simulink model "pendule"  (R2023a)
settings: Solver=VariableStepAuto  StartTime=0.0  StopTime=10.0  RelTol=1e-3
settings Model: Creator=gwr2526  LastModifiedBy=gwr2526

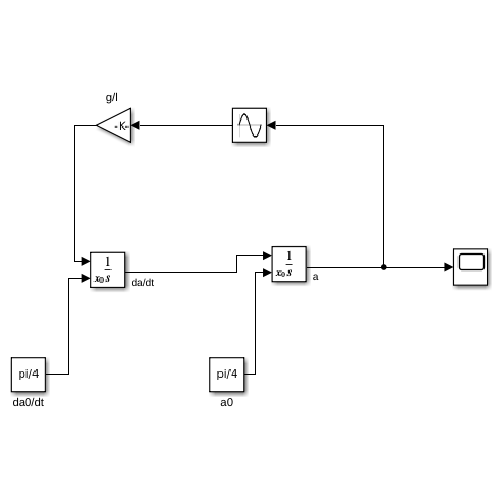
[thumbnail: Simulink's stored preview of the top-level diagram]
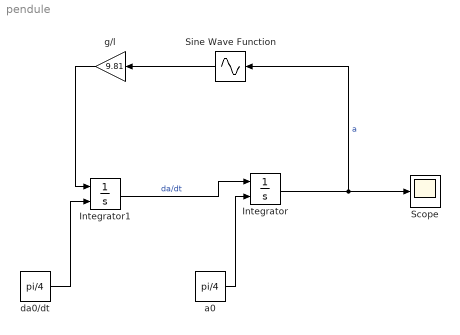
== system pendule ==
  Integrator : Integrator  InitialConditionSource=external
  Integrator1 : Integrator  InitialConditionSource=external
  Scope : Scope
  Sine Wave Function : Sin  TimeSource=Use external signal  SampleTime=0
  a0 : Constant  Value=pi/4
  da0/dt : Constant  Value=pi/4
  "g/l " : Gain  Gain=9.81
  wires:
  Integrator1/1 -> Integrator/1  "da/dt"
  a0/1 -> Integrator/2
  da0/dt/1 -> Integrator1/2
  Integrator/1 -> Sine Wave Function/1, Scope/1  "a"
  "g/l "/1 -> Integrator1/1
  Sine Wave Function/1 -> "g/l "/1
